simulink model "FlexSensor_OpAmp2"  (R2017b)
settings: Solver=VariableStepAuto  StartTime=0.0  StopTime=inf  RelTol=1e-3
libraries: fl_lib x13, nesl_utility x5
settings Model: Creator=root  LastModifiedBy=root

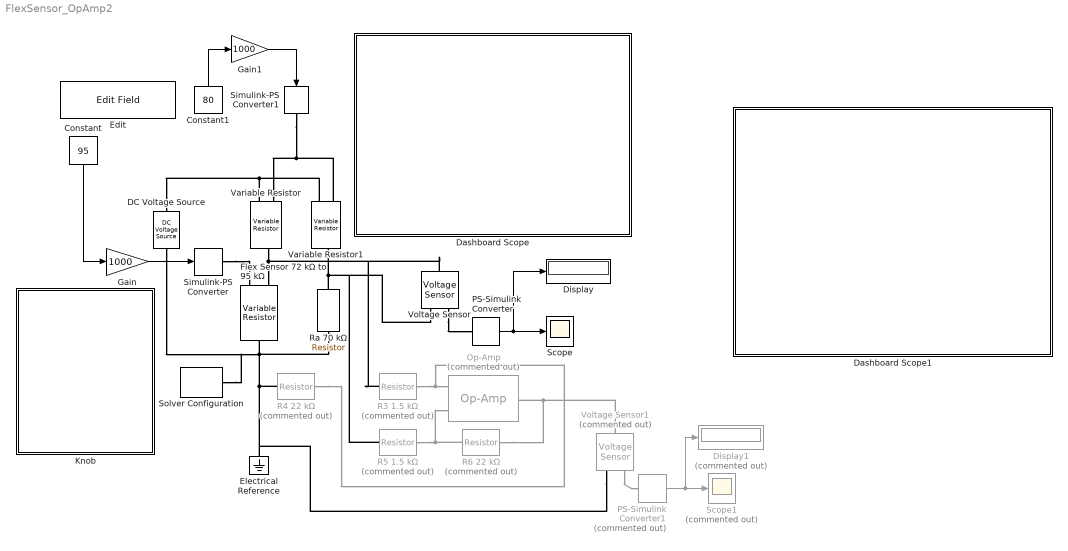
== system FlexSensor_OpAmp2 ==
  Constant : Constant  Value=95
  Constant1 : Constant  Value=80
  DC Voltage Source : fl_lib/Electrical/Electrical Sources/DC Voltage Source  v0=5 V
  Dashboard Scope : Subsystem  DialogController=hmiCreateDDGDialog  IsWebBlock=on  mask(MWDashboardBlock){webBlockId=d9aacbb0-daaa-4d15-a269-d73fdfd00d43, webBlockType=sdiscope, ShowInitialText=on, HMISrcModelName=FlexSensor_OpAmp2}
      mask prompts: webBlockId "WebBlock Id"; webBlockType "WebBlock Type"; HMISrcModelName "Source Model"
      mask help: SimulinkHMI:dialogs:HMIScopeDialogDesc
      mask Help: helpview([docroot '/mapfiles/simulink.map'], 'hmi_scope')
      mask Display:
      | if strcmp(get_param(bdroot(gcb),'BlockDiagramType'), 'library')
      |     image([(matlabroot) '/toolbox/simulink/hmi/icons/DashboardScope.png']);
      | end
  Dashboard Scope1 : Subsystem  DialogController=hmiCreateDDGDialog  IsWebBlock=on  mask(MWDashboardBlock){webBlockId=79fc4c68-e22f-4fd7-a6c3-05ccfefb5409, webBlockType=sdiscope, ShowInitialText=on, HMISrcModelName=FlexSensor_OpAmp2}
      mask prompts: webBlockId "WebBlock Id"; webBlockType "WebBlock Type"; HMISrcModelName "Source Model"
      mask help: SimulinkHMI:dialogs:HMIScopeDialogDesc
      mask Help: helpview([docroot '/mapfiles/simulink.map'], 'hmi_scope')
      mask Display:
      | if strcmp(get_param(bdroot(gcb),'BlockDiagramType'), 'library')
      |     image([(matlabroot) '/toolbox/simulink/hmi/icons/DashboardScope.png']);
      | end
  Display : Display
  Display1 : Display  Commented=on
  Edit : EditField  WebBlockId=7  ModelName=FlexSensor_OpAmp2  LabelPosition=Top  ShowInitialText=off  Alignment=Center
  Electrical Reference : fl_lib/Electrical/Electrical Elements/Electrical Reference
  Flex Sensor 72 kΩ to 95 kΩ : fl_lib/Electrical/Electrical Elements/Variable Resistor  Rmin=72 kOhm  i_specify=off  i_priority=None  i=0 A  i_nominal_specify=off  i_nominal_unit=A  i_nominal_value=1  v_specify=off  v_priority=None  v=0 V  v_nominal_specify=off  v_nominal_unit=V  v_nominal_value=1
  Gain : Gain  Gain=1000
  Gain1 : Gain  Gain=1000
  Knob : Subsystem  DialogController=hmiCreateDDGDialog  IsWebBlock=on  mask(MWDashboardBlock){webBlockId=d0dba7f8-e92f-4e85-9496-0227f963a3eb, webBlockType=continuousknob, ShowInLibBrowser=on, ShowInitialText=on, HMISrcModelName=FlexSensor_OpAmp2}
      mask prompts: webBlockId "WebBlock Id"; webBlockType "WebBlock Type"; HMISrcModelName "Source Model"
      mask help: SimulinkHMI:dialogs:ContinuousKnobDialogDesc
      mask Help: helpview([docroot '/mapfiles/simulink.map'], 'hmi_knob')
      mask Display:
      | if strcmp(get_param(bdroot(gcb),'BlockDiagramType'), 'library')
      |     image([(matlabroot) '/toolbox/simulink/hmi/icons/ContinuousKnob.png']);
      | end
  Op-Amp : fl_lib/Electrical/Electrical Elements/Op-Amp  Commented=on  outI_specify=off  outI_priority=None  outI=0 A  outI_nominal_specify=off  outI_nominal_unit=A  outI_nominal_value=1
  PS-Simulink Converter : nesl_utility/PS-Simulink Converter  PhysicalDomain=network_engine_domain  SubClassName=ps_output  LeftPortType=input  RightPortType=output  PseudoPeriodic=off  Frequencies=[]  Unit=1  AffineConversion=off
  PS-Simulink Converter1 : nesl_utility/PS-Simulink Converter  Commented=on  PhysicalDomain=network_engine_domain  SubClassName=ps_output  LeftPortType=input  RightPortType=output  PseudoPeriodic=off  Frequencies=[]  Unit=1  AffineConversion=off
  R3 1.5 kΩ : fl_lib/Electrical/Electrical Elements/Resistor  Commented=on  R=1.5 kOhm  i_specify=off  i_priority=None  i=0 A  i_nominal_specify=off  i_nominal_unit=A  i_nominal_value=1  v_specify=off  v_priority=None  v=0 V  v_nominal_specify=off  v_nominal_unit=V  v_nominal_value=1
  R4 22 kΩ : fl_lib/Electrical/Electrical Elements/Resistor  Commented=on  R=22 kOhm  i_specify=off  i_priority=None  i=0 A  i_nominal_specify=off  i_nominal_unit=A  i_nominal_value=1  v_specify=off  v_priority=None  v=0 V  v_nominal_specify=off  v_nominal_unit=V  v_nominal_value=1
  R5 1.5 kΩ : fl_lib/Electrical/Electrical Elements/Resistor  Commented=on  R=1.5 kOhm  i_specify=off  i_priority=None  i=0 A  i_nominal_specify=off  i_nominal_unit=A  i_nominal_value=1  v_specify=off  v_priority=None  v=0 V  v_nominal_specify=off  v_nominal_unit=V  v_nominal_value=1
  R6 22 kΩ : fl_lib/Electrical/Electrical Elements/Resistor  Commented=on  R=22 kOhm  i_specify=off  i_priority=None  i=0 A  i_nominal_specify=off  i_nominal_unit=A  i_nominal_value=1  v_specify=off  v_priority=None  v=0 V  v_nominal_specify=off  v_nominal_unit=V  v_nominal_value=1
  Ra 70 kΩ : fl_lib/Electrical/Electrical Elements/Resistor  R=70 kOhm  i_specify=off  i_priority=None  i=0 A  i_nominal_specify=off  i_nominal_unit=A  i_nominal_value=1  v_specify=off  v_priority=None  v=0 V  v_nominal_specify=off  v_nominal_unit=V  v_nominal_value=1
  Scope : Scope
  Scope1 : Scope  Commented=on
  Simulink-PS Converter : nesl_utility/Simulink-PS Converter  PhysicalDomain=network_engine_domain  SubClassName=ps_input  LeftPortType=input  RightPortType=output  PseudoPeriodic=off  Frequencies=[]  NoiseDistribution=none  NoiseParameters=[]  Unit=1  AffineConversion=off  FilteringAndDerivatives=provide  SimscapeFilterOrder=1  InputFilterTimeConstant=0.001  UdotUserProvided=0
  Simulink-PS Converter1 : nesl_utility/Simulink-PS Converter  PhysicalDomain=network_engine_domain  SubClassName=ps_input  LeftPortType=input  RightPortType=output  PseudoPeriodic=off  Frequencies=[]  NoiseDistribution=none  NoiseParameters=[]  Unit=1  AffineConversion=off  FilteringAndDerivatives=provide  SimscapeFilterOrder=1  InputFilterTimeConstant=0.001  UdotUserProvided=0
  Solver Configuration : nesl_utility/Solver Configuration  PhysicalDomain=network_engine_domain  SubClassName=solver  LeftPortType=input  RightPortType=generic  Accelerate=off  Tones=[]  Harmonics=[]  SimulateNoise=off  Profile=off  UseLocalSampling=off  EnableSwitchedLinearOptims=on  FrequencyDomain=off  UseCCode=off  RelTol=0.001  AbsTol=1e-06  MinStep=1e-09  ToWorkspace=off  RevertToSquareIcSolve=off  NumHomotopyIterations=100  PhasorMode=off  PhasorModeNumHarmonics=1  DoDC=off  ResidualTolerance=1e-09  UseLocalSolver=off  LocalSolverChoice=NE_BACKWARD_EULER_ADVANCER  LocalSolverSampleTime=0.001  DoFixedCost=off  MaxNonlinIter=3  MaxModeIter=2  LinearAlgebra=Sparse  DelaysMemoryBudget=1024  AutomaticFiltering=on  FilteringTimeConstant=0.001
  Variable Resistor : fl_lib/Electrical/Electrical Elements/Variable Resistor  Rmin=0 Ohm  i_specify=off  i_priority=None  i=0 A  i_nominal_specify=off  i_nominal_unit=A  i_nominal_value=1  v_specify=off  v_priority=None  v=0 V  v_nominal_specify=off  v_nominal_unit=V  v_nominal_value=1
  Variable Resistor1 : fl_lib/Electrical/Electrical Elements/Variable Resistor  Rmin=0 Ohm  i_specify=off  i_priority=None  i=0 A  i_nominal_specify=off  i_nominal_unit=A  i_nominal_value=1  v_specify=off  v_priority=None  v=0 V  v_nominal_specify=off  v_nominal_unit=V  v_nominal_value=1
  Voltage Sensor : fl_lib/Electrical/Electrical Sensors/Voltage Sensor
  Voltage Sensor1 : fl_lib/Electrical/Electrical Sensors/Voltage Sensor  Commented=on
  wires:
  Gain1/1 -> Simulink-PS Converter1/1
  Constant1/1 -> Gain1/1
  Constant/1 -> Gain/1
  Gain/1 -> Simulink-PS Converter/1
  PS-Simulink Converter/1 -> Display/1, Scope/1
  PS-Simulink Converter1/1 -> Display1/1, Scope1/1
  connections:
  Simulink-PS Converter1/RConn1 -- Variable Resistor/LConn1 -- Variable Resistor1/LConn1
  Variable Resistor/RConn1 -- R3 1.5 kΩ/RConn1 -- Voltage Sensor/LConn1 -- Flex Sensor 72 kΩ to 95 kΩ/LConn2
  Variable Resistor/LConn2 -- DC Voltage Source/LConn1 -- Variable Resistor1/LConn2
  Ra 70 kΩ/LConn1 -- R5 1.5 kΩ/RConn1 -- Voltage Sensor/RConn2 -- Variable Resistor1/RConn1
  Ra 70 kΩ/RConn1 -- Electrical Reference/LConn1 -- Voltage Sensor1/RConn2 -- R4 22 kΩ/RConn1 -- Solver Configuration/RConn1 -- DC Voltage Source/RConn1 -- Flex Sensor 72 kΩ to 95 kΩ/RConn1
  Simulink-PS Converter/RConn1 -- Flex Sensor 72 kΩ to 95 kΩ/LConn1
  Voltage Sensor/RConn1 -- PS-Simulink Converter/LConn1
  R6 22 kΩ/LConn1 -- Op-Amp/RConn1 -- Voltage Sensor1/LConn1
  R6 22 kΩ/RConn1 -- Op-Amp/LConn2 -- R5 1.5 kΩ/LConn1
  R3 1.5 kΩ/LConn1 -- R4 22 kΩ/LConn1 -- Op-Amp/LConn1
  Voltage Sensor1/RConn1 -- PS-Simulink Converter1/LConn1

== system FlexSensor_OpAmp2/Dashboard Scope ==

== system FlexSensor_OpAmp2/Dashboard Scope1 ==

== system FlexSensor_OpAmp2/Knob ==
